simulink model "model_autopilot"  (R2018b)
settings: Solver=VariableStepAuto  StartTime=0.0  StopTime=sim_time  RelTol=1e-3
values from neighbouring files (symbols this model uses):
  a_phi_1 = 2.87    [A2_Part1.m]    (also in A2_Part1_med2e.m = -0.65)
  a_phi_2 = -0.65    [A2_Part1.m]    (also in A2_Part1_med2e.m = 2.87)
  d = 1.5*pi/180    (= 0.0261799387799)    [A2_Part1.m]    (also in A2_Part1_med2e.m = 1.5; A2_part1_2e_jalla.m)
  g = 9.81    [A2_Part1_med2e.m]    (also in A2_part1_2e_jalla.m)
  k_d_phi = (2 * zeta_phi * omega_n_phi - a_phi_1)/a_phi_2    [A2_Part1.m]    (also in A2_Part1_med2e.m = 2 * zeta_phi * omega_n_phi/a_phi_2; A2_part1_2e_jalla.m = (2*seta_phi*omega_phi - a_1)/a_2)
  k_i_chi = omega_n_chi^2 * V_g/g    [A2_Part1.m]    (also in A2_Part1_med2e.m; A2_part1_2e_jalla.m = (omega_chi^2)*V_a/g)
  k_p_chi = 2 * zeta_chi * omega_n_chi * V_g/g    [A2_Part1.m]    (also in A2_Part1_med2e.m; A2_part1_2e_jalla.m = 2*seta_chi*omega_chi*V_a/g)
  k_p_phi = delta_a_max/e_phi_max * sign(a_phi_2)    [A2_Part1.m]    (also in A2_Part1_med2e.m; A2_part1_2e_jalla.m = -2)
  V_g = V_a    [A2_Part1.m]    (also in A2_Part1_med2e.m)
libraries: simulink_extras x3
settings Model: Creator=gustavoo  LastModifiedBy=Magne Sirnes
settings DataIOCC: ReturnWorkspaceOutputs=on

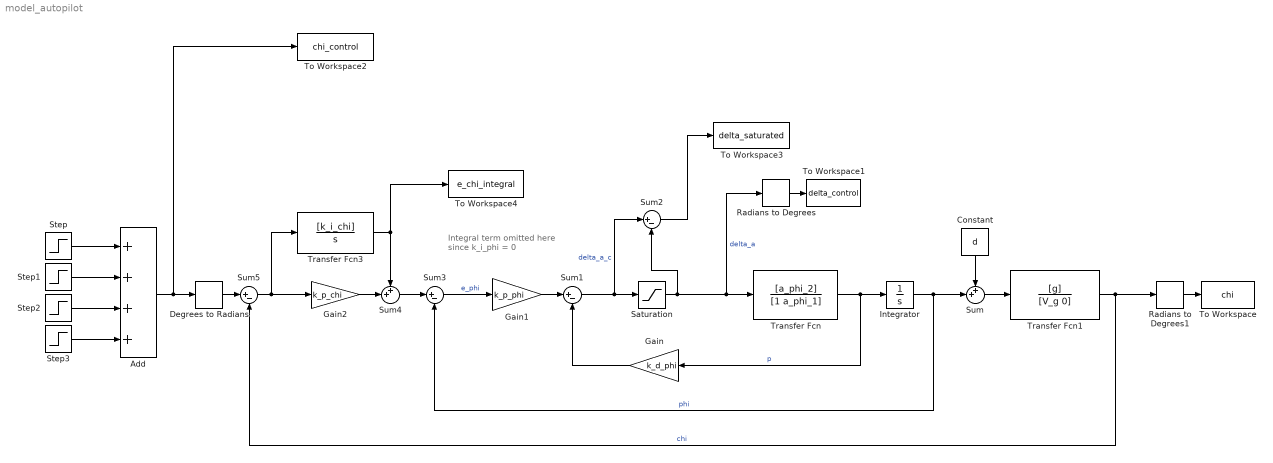
== system model_autopilot ==
  note: Integral term omitted here
      | since k_i_phi = 0
  Add : Sum  Inputs=++++
  Constant : Constant  Value=d
  Degrees to Radians : simulink_extras/Transformations/Degrees to Radians
  Gain : Gain  Gain=k_d_phi
  Gain1 : Gain  Gain=k_p_phi
  Gain2 : Gain  Gain=k_p_chi
  Integrator : Integrator
  Radians to Degrees : simulink_extras/Transformations/Radians to Degrees
  Radians to Degrees1 : simulink_extras/Transformations/Radians to Degrees
  Saturation : Saturate  UpperLimit=pi/6  LowerLimit=-pi/6
  Step : Step  Time=100  After=7.5  SampleTime=0
  Step1 : Step  Time=150  After=7.5  SampleTime=0
  Step2 : Step  Time=250  After=-15  SampleTime=0
  Step3 : Step  Time=300  After=0  SampleTime=0
  Sum : Sum  Inputs=++|
  Sum{1..3,5} (4 alike) : Sum  Inputs=|+-
  Sum4 : Sum  Inputs=++|
  To Workspace : ToWorkspace  VariableName=chi  SaveFormat=Timeseries  SampleTime=-1
  To Workspace1 : ToWorkspace  VariableName=delta_control  SaveFormat=Timeseries  SampleTime=-1
  To Workspace2 : ToWorkspace  VariableName=chi_control  SaveFormat=Timeseries  SampleTime=-1
  To Workspace3 : ToWorkspace  VariableName=delta_saturated  SaveFormat=Timeseries  SampleTime=-1
  To Workspace4 : ToWorkspace  VariableName=e_chi_integral  SaveFormat=Timeseries  SampleTime=-1
  Transfer Fcn : TransferFcn  Numerator=[a_phi_2]  Denominator=[1 a_phi_1]
  Transfer Fcn1 : TransferFcn  Numerator=[g]  Denominator=[V_g 0]
  Transfer Fcn3 : TransferFcn  Numerator=[k_i_chi]  Denominator=[1 0]
  wires:
  Sum/1 -> Transfer Fcn1/1
  Integrator/1 -> Sum/2, Sum3/2  "phi"
  Constant/1 -> Sum/1
  Transfer Fcn/1 -> Integrator/1, Gain/1  "p"
  Sum1/1 -> Sum2/1, Saturation/1  "delta_a_c"
  Gain/1 -> Sum1/2
  Gain1/1 -> Sum1/1
  Sum3/1 -> Gain1/1  "e_phi"
  Sum4/1 -> Sum3/1
  Gain2/1 -> Sum4/2
  Transfer Fcn3/1 -> Sum4/1, To Workspace4/1
  Sum5/1 -> Transfer Fcn3/1, Gain2/1
  Transfer Fcn1/1 -> Sum5/2, Radians to Degrees1/1  "chi"
  Saturation/1 -> Transfer Fcn/1, Radians to Degrees/1, Sum2/2  "delta_a"
  Degrees to Radians/1 -> Sum5/1
  Step1/1 -> Add/2
  Step/1 -> Add/1
  Step3/1 -> Add/4
  Step2/1 -> Add/3
  Add/1 -> To Workspace2/1, Degrees to Radians/1
  Radians to Degrees1/1 -> To Workspace/1
  Radians to Degrees/1 -> To Workspace1/1
  Sum2/1 -> To Workspace3/1
